simulink model "ARDroneReplayKalmanRollBias"  (R2023b)
settings: Solver=ode1  StartTime=0.0  StopTime=54.2150  FixedStep=sampleTime  RelTol=1e-3
values from neighbouring files (symbols this model uses):
  A = 0    [calcKalmanGain_pitch_only.m]    (also in simKalmanSettingsPitch.m = [0]; simKalmanSettingsPitchBias.m = [0 -1; 0 0]; simKalmanSettingsRoll.m = [0]; simKalmanSettingsRollBias.m = [[0 -1]; [0 0]])
  B = 1    [calcKalmanGain_pitch_only.m]    (also in simKalmanSettingsPitch.m = [1]; simKalmanSettingsPitchBias.m = [1; 0]; simKalmanSettingsRoll.m = [1]; simKalmanSettingsRollBias.m = [1; 0])
  C = 1    [calcKalmanGain_pitch_only.m]    (also in simKalmanSettingsPitch.m = [1]; simKalmanSettingsPitchBias.m = [1 0]; simKalmanSettingsRoll.m = [1]; simKalmanSettingsRollBias.m = [1 0])
  D = 0    [calcKalmanGain_pitch_only.m]    (also in simKalmanSettingsPitch.m = [0]; simKalmanSettingsPitchBias.m; simKalmanSettingsRoll.m = [0]; simKalmanSettingsRollBias.m)
  R = 1    [calcKalmanGain_pitch_only.m]    (also in simKalmanSettingsPitch.m = 0.116166; simKalmanSettingsPitchBias.m = 100*Q(1,1); simKalmanSettingsRoll.m = 0.025232; simKalmanSettingsRollBias.m = Q(1,1)*1000)
  sampleTime = 1/200    (= 0.005)    [setupReplay.m]    (also in setupReplayKalmanPitch.m; setupReplayKalmanPitchBias.m; setupReplayKalmanRoll.m; setupReplayKalmanRollBias.m)
undefined symbols (not defined in the file or in its folder): Continuous, meanAcce3, Time
libraries: ARBlocks x2, ctrlSharedLib x1
settings Model: ExtModeTrigDuration=100000  Creator=Paul  LastModifiedBy=André
settings SolverCC: AlgebraicLoopSolver=TrustRegion  AutoInsertRateTranBlk=on
settings DataIOCC: LimitDataPoints=on  SaveFormat=Array  SignalLoggingSaveFormat=ModelDataLogs  ReturnWorkspaceOutputs=off  TimeSaveName=time
settings OptimizationCC: ExpressionDepthLimit=2147483647  InitFltsAndDblsToZero=on
settings DebuggingCC: UnderspecifiedInitializationDetection=Classic  MergeDetectMultiDrivingBlocksExec=none  SolverPrmCheckMsg=warning  FcnCallInpInsideContextMsg=warning  UnconnectedInputMsg=warning  UnconnectedOutputMsg=warning  UnconnectedLineMsg=warning  StateNameClashWarn=warning  SFUnexpectedBacktrackingDiag=warning  SFNoUnconditionalDefaultTransitionDiag=warning  SFExecutionAtInitializationDiag=none  ArithmeticOperatorsInVariantConditions=warning
settings HardwareCC: ProdBitPerLong=64  ProdHWDeviceType=Intel->x86-64 (Linux 64)
settings ModelReferenceCC: EnableRefExpFcnMdlSchedulingChecks=on  PropagateSignalLabelsOutOfModel=off
settings SFSimCC: SimUseLocalCustomCode=off  CustomCodeUndefinedFunction=UseInterfaceOnly
settings RTWCC: Description=Simulink Desktop Real-Time  SystemTargetFile=sldrt.tlc  TemplateMakefile=sldrt.tmf  RTWUseLocalCustomCode=off  RTWCompilerOptimization=on
settings CodeAppCC: MaxIdLength=95  StateflowObjectComments=on
settings SimulinkDesktopRealTimeCC: TargetLibSuffix=_sldrt.a  TargetPreCompLibLocation=C:\Program Files\MATLAB\R2023b\toolbox\sldrt\lib\win64  TargetLangStandard=C89/C90 (ANSI)  SupportVariableSizeSignals=off
settings ConfigComp: CovMetricSettings=dw  CovSaveCumulativeToWorkspaceVar=on  CovSaveSingleToWorkspaceVar=on  CovExternalEMLEnable=off

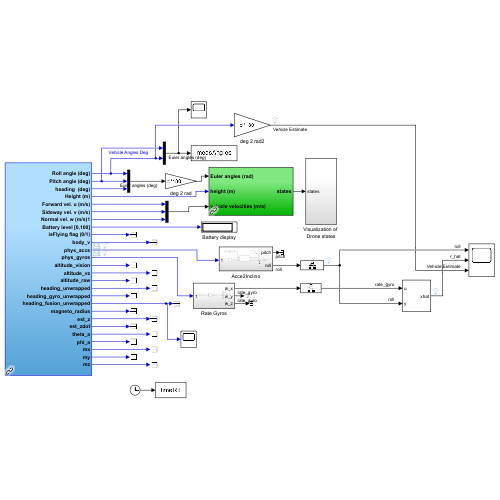
[thumbnail: Simulink's stored preview of the top-level diagram]
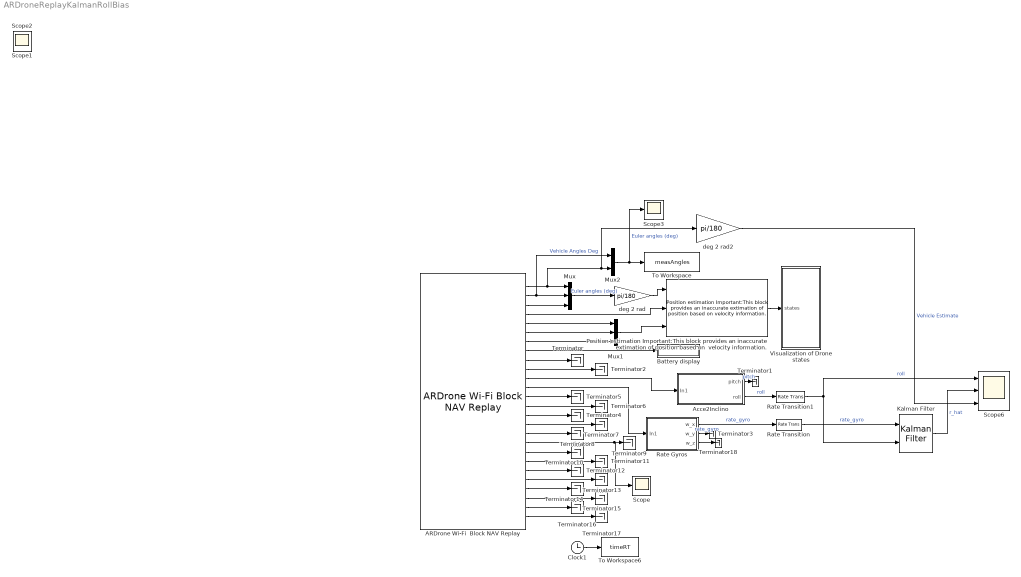
== system ARDroneReplayKalmanRollBias ==
  ARDrone Wi-Fi  Block NAV Replay : ARBlocks/ARDrone Wi-Fi  Block NAV Replay  SystemSampleTime=-1  VariantActivationTime=update diagram  AllowFlexibleInterface=on  Latency=0  AutoFrameSizeCalculation=off
  Acce2Inclino : Subsystem
  Battery display : Display
  Clock1 : Clock
  Kalman Filter : ctrlSharedLib/Kalman Filter  TimeDomain=Continuous-Time  UseCurrentEstimator=on  ModelSource=Individual A, B, C, D matrices  ModelSourceVariable=ss(0.95,1,1,0,1)  A=A  B=B  C=C  D=D  NumberOfStates=1  NumberOfInputs=1  NumberOfOutputs=1  InitialEstimateSource=Dialog  X0=0  P0=10  UseK=off  UseGH=off  NumberOfProcessNoiseInputs=1  G=1  TimeInvariantG=on  H=0  TimeInvariantH=on  Q=Q  TimeInvariantQ=on  R=R  TimeInvariantR=on  N=0  TimeInvariantN=on  AddInputPort=on  AddEnablePort=off  OutputEstimatedY=off  OutputP=off  Ts=-1
  Mux : Mux  Inputs=3
  Mux1 : Mux  Inputs=3
  Mux2 : Mux  Inputs=2
  "Position estimation Important:This block provides an inaccurate extimation of position based on  velocity information. " : ARBlocks/Position estimation Important:This block provides an  inaccurate extimation of position  based on  velocity information.   SystemSampleTime=-1  VariantActivationTime=update diagram  AllowFlexibleInterface=on  Latency=0  AutoFrameSizeCalculation=off
  Rate Gyros : Subsystem
  Rate Transition : RateTransition  OutPortSampleTime=0
  Rate Transition1 : RateTransition  OutPortSampleTime=0
  Scope{,1..3} (4 alike) : Scope
  Scope6 : Scope  NumInputPorts=3
  Terminator{,1..18} (19 alike) : Terminator
  To Workspace : ToWorkspace  VariableName=measAngles  SaveFormat=Structure With Time  SampleTime=-1
  To Workspace6 : ToWorkspace  VariableName=timeRT  SampleTime=sampleTime
  Visualization of Drone states : Subsystem
  deg 2 rad : Gain  Gain=pi/180
  deg 2 rad2 : Gain  Gain=pi/180
  wires:
  ARDrone Wi-Fi  Block NAV Replay/1 -> deg 2 rad2/1, Mux2/2, Mux/1
  ARDrone Wi-Fi  Block NAV Replay/2 -> Mux2/1, Mux/2  "Vehicle Angles Deg"
  ARDrone Wi-Fi  Block NAV Replay/5 -> Mux1/1
  ARDrone Wi-Fi  Block NAV Replay/6 -> Mux1/2
  ARDrone Wi-Fi  Block NAV Replay/7 -> Mux1/3
  Mux/1 -> deg 2 rad/1  "Euler angles (deg)"
  ARDrone Wi-Fi  Block NAV Replay/8 -> Battery display/1
  "Position estimation Important:This block provides an inaccurate extimation of position based on  velocity information. "/1 -> Visualization of Drone states/1(states)
  deg 2 rad/1 -> "Position estimation Important:This block provides an inaccurate extimation of position based on  velocity information. "/1
  ARDrone Wi-Fi  Block NAV Replay/4 -> "Position estimation Important:This block provides an inaccurate extimation of position based on  velocity information. "/2
  Mux1/1 -> "Position estimation Important:This block provides an inaccurate extimation of position based on  velocity information. "/3
  ARDrone Wi-Fi  Block NAV Replay/3 -> Mux/3
  ARDrone Wi-Fi  Block NAV Replay/9 -> Terminator/1
  Clock1/1 -> To Workspace6/1
  ARDrone Wi-Fi  Block NAV Replay/15 -> Terminator4/1
  ARDrone Wi-Fi  Block NAV Replay/10 -> Terminator2/1
  ARDrone Wi-Fi  Block NAV Replay/13 -> Terminator5/1
  ARDrone Wi-Fi  Block NAV Replay/14 -> Terminator6/1
  ARDrone Wi-Fi  Block NAV Replay/17 -> Terminator8/1
  ARDrone Wi-Fi  Block NAV Replay/16 -> Terminator7/1
  ARDrone Wi-Fi  Block NAV Replay/19 -> Terminator10/1
  ARDrone Wi-Fi  Block NAV Replay/18 -> Scope/1, Terminator9/1
  ARDrone Wi-Fi  Block NAV Replay/21 -> Terminator12/1
  ARDrone Wi-Fi  Block NAV Replay/20 -> Terminator11/1
  ARDrone Wi-Fi  Block NAV Replay/23 -> Terminator14/1
  ARDrone Wi-Fi  Block NAV Replay/22 -> Terminator13/1
  ARDrone Wi-Fi  Block NAV Replay/25 -> Terminator16/1
  ARDrone Wi-Fi  Block NAV Replay/24 -> Terminator15/1
  ARDrone Wi-Fi  Block NAV Replay/26 -> Terminator17/1
  Mux2/1 -> Scope3/1, To Workspace/1  "Euler angles (deg)"
  ARDrone Wi-Fi  Block NAV Replay/11 -> Acce2Inclino/1(In1)
  ARDrone Wi-Fi  Block NAV Replay/12 -> Rate Gyros/1(In1)
  Rate Gyros/3(w_z) -> Terminator18/1
  Acce2Inclino/1(pitch) -> Terminator1/1  "pitch"
  Rate Gyros/2(w_y) -> Terminator3/1  "rate_gyro"
  Rate Transition/1 -> Kalman Filter/1  "rate_gyro"
  deg 2 rad2/1 -> Scope6/3  "Vehicle Estimate"
  Kalman Filter/1 -> Scope6/2  "r_hat"
  Rate Transition1/1 -> Kalman Filter/2, Scope6/1  "roll"
  Acce2Inclino/2(roll) -> Rate Transition1/1  "roll"
  Rate Gyros/1(w_x) -> Rate Transition/1  "rate_gyro"

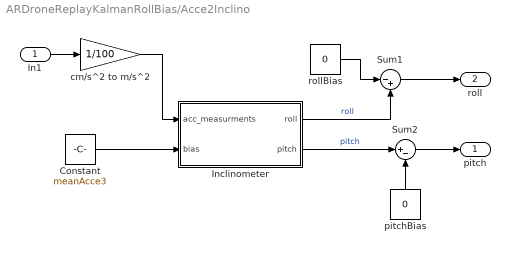
== system ARDroneReplayKalmanRollBias/Acce2Inclino ==
  In1 : Inport
  Constant : Constant  Value=meanAcce3  VectorParams1D=off
  Inclinometer : MATLAB Function  TreatAsAtomicUnit=on
  Sum1 : Sum  Inputs=|-+
  Sum2 : Sum  Inputs=|+-
  cm/s^2 to m/s^2 : Gain  Gain=1/100
  pitchBias : Constant  Value=0
  rollBias : Constant  Value=0
  pitch : Outport
  roll : Outport  Port=2
  wires:
  Sum2/1 -> pitch/1
  Inclinometer/2(pitch) -> Sum2/1  "pitch"
  Inclinometer/1(roll) -> Sum1/2  "roll"
  cm/s^2 to m/s^2/1 -> Inclinometer/1(acc_measurments)
  pitchBias/1 -> Sum2/2
  In1/1 -> cm/s^2 to m/s^2/1
  Sum1/1 -> roll/1
  rollBias/1 -> Sum1/1
  Constant/1 -> Inclinometer/2(bias)

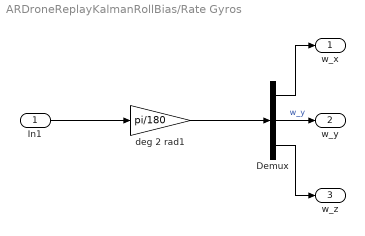
== system ARDroneReplayKalmanRollBias/Rate Gyros ==
  In1 : Inport
  Demux : Demux  Outputs=3
  deg 2 rad1 : Gain  Gain=pi/180
  w_x : Outport
  w_y : Outport  Port=2
  w_z : Outport  Port=3
  wires:
  Demux/1 -> w_x/1
  deg 2 rad1/1 -> Demux/1
  In1/1 -> deg 2 rad1/1
  Demux/2 -> w_y/1  "w_y"
  Demux/3 -> w_z/1

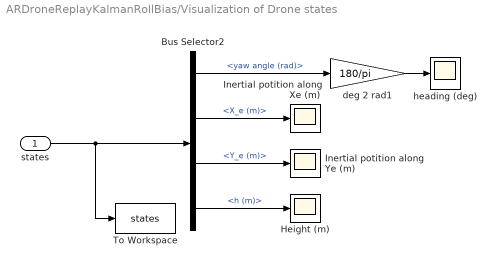
== system ARDroneReplayKalmanRollBias/Visualization of Drone states ==
  states : Inport
  Bus Selector2 : BusSelector  OutputSignals=yaw angle (rad),X_e (m),Y_e (m),h (m)
  Height (m) : Scope
  Inertial potition along Xe (m) : Scope
  Inertial potition along Ye (m) : Scope
  To Workspace : ToWorkspace  VariableName=states  SaveFormat=Structure With Time  SampleTime=-1
  deg 2 rad1 : Gain  Gain=180/pi
  heading (deg) : Scope
  wires:
  states/1 -> To Workspace/1, Bus Selector2/1
  Bus Selector2/1 -> deg 2 rad1/1  "<yaw angle (rad)>"
  Bus Selector2/2 -> Inertial potition along Xe (m)/1  "<X_e (m)>"
  Bus Selector2/3 -> Inertial potition along Ye (m)/1  "<Y_e (m)>"
  Bus Selector2/4 -> Height (m)/1  "<h (m)>"
  deg 2 rad1/1 -> heading (deg)/1

== matlab function ARDroneReplayKalmanRollBias/Acce2Inclino/Inclinometer ==
  data: acc_measurments input; roll output; pitch output; bias input
function [roll, pitch] = fcn(acc_measurments, bias)
ax = acc_measurments(1) - bias(1);
ay = acc_measurments(2) - bias(2);
az = acc_measurments(3) - (bias(3)+9.8);

% ax = acc_measurments(1);
% ay = acc_measurments(2);
% az = acc_measurments(3);


ag = sqrt(ax*ax + ay*ay + az*az);
if ag == 0 && az == 0
    roll = 0;
    pitch = 0;
    return
elseif ag == 0
    pitch = 0;
    roll = atan(ay/az);
elseif az == 0
    roll = 0;
    pitch = asin(ax/ag);
else
    roll = atan(ay/az);
    pitch = asin(ax/ag);
end
